simulink subsystem "subsystem_amplitude_modulation_simplified"  (R2022a)
settings: Solver=VariableStepAuto  StartTime=0.0  StopTime=10.0  RelTol=1e-3
undefined symbols (not defined in the file): cos_amp, cos_center, ref_angle, rel_diff, timescale
libraries: neuromorphic_blocks x10
settings Model: Creator=chris  LastModifiedBy=chris

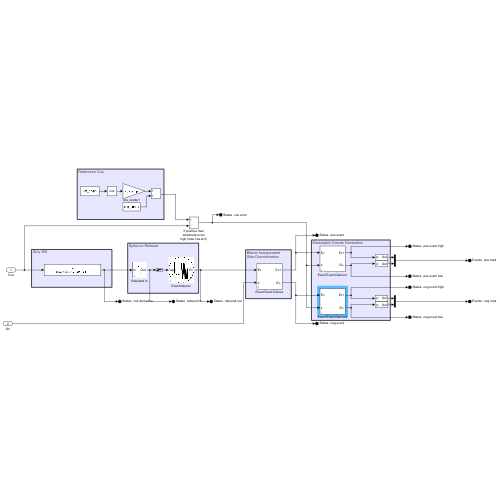
[thumbnail: Simulink's stored preview of the top-level diagram]
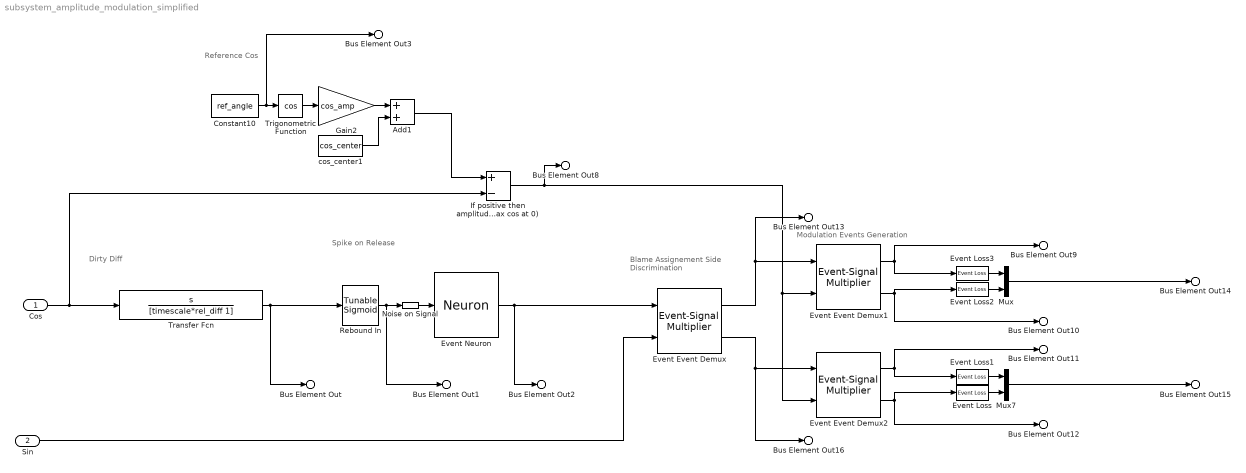
== system subsystem_amplitude_modulation_simplified ==
  note: Dirty Diff
  note: Spike on Release
  note: Reference Cos
  note: Blame Assignement
      | Side Discrimination
  note: Modulation Events Generation
  Cos : Inport
  Sin : Inport  Port=2
  Add1 : Sum
  Constant10 : Constant  Value=ref_angle  LockScale=on
  Event Event Demux : neuromorphic_blocks/Auxiliary Blocks/Event-Signal Multiplier  symmetric_box=off  dsyn_signal_pos=0.0  dsyn_signal_neg=0.0  dsyn_signal_neg_save=0.0  gain_signal_pos=100  gain_signal_neg=100  gain_signal_neg_save=100  input=Events  gsyn_pos=20  gsyn_neg=20  gsyn_neg_save=20  dsyn_event_pos=10  dsyn_event_neg=10  dsyn_event_neg_save=10  gain_event_pos=20  gain_event_neg=20  gain_event_neg_save=20
      settings: SourceProductName=NeurCont Toolbox
  Event Event Demux1 : neuromorphic_blocks/Auxiliary Blocks/Event-Signal Multiplier  symmetric_box=off  dsyn_signal_pos=0  dsyn_signal_neg=0  dsyn_signal_neg_save=0  gain_signal_pos=-100  gain_signal_neg=-100  gain_signal_neg_save=100  input=Events  gsyn_pos=20  gsyn_neg=20  gsyn_neg_save=20  dsyn_event_pos=10  dsyn_event_neg=10  dsyn_event_neg_save=10  gain_event_pos=20  gain_event_neg=20  gain_event_neg_save=20
      settings: SourceProductName=NeurCont Toolbox
  Event Event Demux2 : neuromorphic_blocks/Auxiliary Blocks/Event-Signal Multiplier  symmetric_box=off  dsyn_signal_pos=0  dsyn_signal_neg=0  dsyn_signal_neg_save=0  gain_signal_pos=-100  gain_signal_neg=-100  gain_signal_neg_save=100  input=Events  gsyn_pos=20  gsyn_neg=20  gsyn_neg_save=20  dsyn_event_pos=10  dsyn_event_neg=10  dsyn_event_neg_save=10  gain_event_pos=20  gain_event_neg=20  gain_event_neg_save=20
      settings: SourceProductName=NeurCont Toolbox
  Event Loss{,1..3} (4 alike) : neuromorphic_blocks/Events Transmission Blocks/Event Loss  loss_prob=prob_event_loss  seed=-1  seed_mem=randi([0, 100000])
      settings: SourceProductName=Neuromorphic Toolbox
  Event Neuron : neuromorphic_blocks/Neural Blocks/Neuron  gfm_source=Internal  gfm=3  gsp_source=Internal  gsp=10  gsm_source=Internal  gsm=0  gup_source=Internal  gup=0  gum_source=Internal  gum=0  dfm=0  dsp=0.5  dsm=-0.5  dup=-0.5  dum=-1.0  mfm=1.0  msp=1.0  msm=1.0  mup=1.0  mum=1.0  timescale=timescale  rel_membrane=0.1  rel_fast=0.1  rel_slow=4  rel_ultraslow=200  Iapp_base=0  V0=-1.2  tresh=0  output=Events
      settings: SourceProductName=Neuromorphic Toolbox
  Gain2 : Gain  Gain=cos_amp
  If positive then amplitude is too high (max cos at 0) : Sum  Inputs=+-
  Mux : Mux  Inputs=2
  Mux7 : Mux  Inputs=2
  Noise on Signal : neuromorphic_blocks/Auxiliary Blocks/Noise on Signal  noise_pwr=noisePwr  timescale=timescale  rel_timescale=rel_noise  seed=-1  seed_mem=randi([0, 100000])
      settings: SourceProductName=NeurCont Toolbox
  Rebound In : neuromorphic_blocks/Tunable Sigmoid  nonlinearity_type=Sigmoid  gain_source=Internal  gain=-1.5  bias=5  slope=-100
      settings: SourceProductName=Neuromorphic Toolbox
  Transfer Fcn : TransferFcn  Numerator=[1 0]  Denominator=[timescale*rel_diff 1]
  Trigonometric Function : Trigonometry  Operator=cos
  cos_center1 : Constant  Value=cos_center
  Bus Element Out14 : Outport  PortName=Events  Element=pos mod
  Bus Element Out15 : Outport  PortName=Events  Element=neg mod
  Bus Element Out9 : Outport  Port=2  PortName=States  Element=pos event high
  Bus Element Out10 : Outport  Port=2  PortName=States  Element=pos event low
  Bus Element Out11 : Outport  Port=2  PortName=States  Element=neg event high
  Bus Element Out12 : Outport  Port=2  PortName=States  Element=neg event low
  Bus Element Out : Outport  Port=2  PortName=States  Element=cos derivative
  Bus Element Out1 : Outport  Port=2  PortName=States  Element=rebound in
  Bus Element Out2 : Outport  Port=2  PortName=States  Element=rebound out
  Bus Element Out8 : Outport  Port=2  PortName=States  Element=cos error
  Bus Element Out13 : Outport  Port=2  PortName=States  Element=pos event
  Bus Element Out16 : Outport  Port=2  PortName=States  Element=neg event
  Bus Element Out3 : Outport  Port=2  PortName=States  Element=ref angle
  wires:
  Trigonometric Function/1 -> Gain2/1
  If positive then amplitude is too high (max cos at 0)/1 -> Event Event Demux1/2, Event Event Demux2/2, Bus Element Out8/1
  Event Neuron/1 -> Bus Element Out2/1, Event Event Demux/1
  Cos/1 -> If positive then amplitude is too high (max cos at 0)/2, Transfer Fcn/1
  cos_center1/1 -> Add1/2
  Transfer Fcn/1 -> Rebound In/1, Bus Element Out/1
  Rebound In/1 -> Bus Element Out1/1, Noise on Signal/1
  Sin/1 -> Event Event Demux/2
  Gain2/1 -> Add1/1
  Mux7/1 -> Bus Element Out15/1
  Mux/1 -> Bus Element Out14/1
  Event Event Demux2/2 -> Bus Element Out12/1, Event Loss/1
  Event Loss/1 -> Mux7/2
  Event Event Demux2/1 -> Bus Element Out11/1, Event Loss1/1
  Event Loss1/1 -> Mux7/1
  Event Event Demux1/1 -> Bus Element Out9/1, Event Loss3/1
  Event Event Demux1/2 -> Bus Element Out10/1, Event Loss2/1
  Event Loss3/1 -> Mux/1
  Event Loss2/1 -> Mux/2
  Noise on Signal/1 -> Event Neuron/1
  Event Event Demux/2 -> Bus Element Out16/1, Event Event Demux2/1
  Event Event Demux/1 -> Bus Element Out13/1, Event Event Demux1/1
  Add1/1 -> If positive then amplitude is too high (max cos at 0)/1
  Constant10/1 -> Trigonometric Function/1, Bus Element Out3/1
